simulink library "INT_Fans_trq"  (R2016b)
settings: Solver=VariableStepAuto  StartTime=0.0  StopTime=10.0  RelTol=1e-3
settings Model: Creator=xinchangran  LastModifiedBy=xinchangran

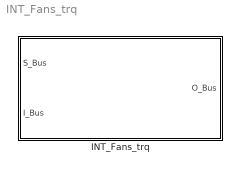
== system INT_Fans_trq ==
  INT_Fans_trq : Subsystem

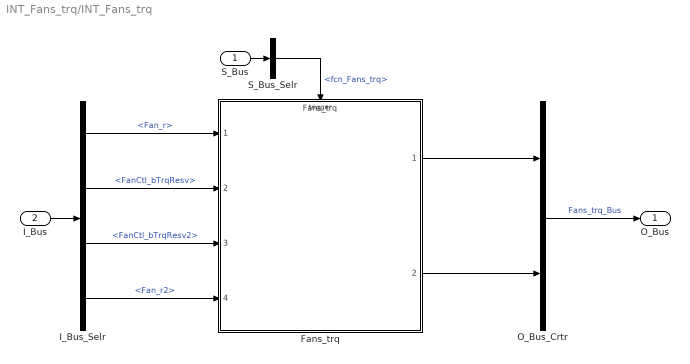
== system INT_Fans_trq/INT_Fans_trq ==
  S_Bus : Inport
  I_Bus : Inport  Port=2
  Fans_trq : ModelReference  ModelNameDialog=Fans_trq  SimulationMode=Normal  ModelReferenceVersion=1.16  TriggerPortName=function  TriggerPortTriggerType=function-call  TriggerPortStatesWhenEnabling=held
  I_Bus_Selr : BusSelector  OutputSignals=Fan_r,FanCtl_bTrqResv,FanCtl_bTrqResv2,Fan_r2
  O_Bus_Crtr : BusCreator  Inputs=2
  S_Bus_Selr : BusSelector  OutputSignals=fcn_Fans_trq
  O_Bus : Outport
  wires:
  S_Bus_Selr/1 -> Fans_trq/Trigger  "<fcn_Fans_trq>"
  S_Bus/1 -> S_Bus_Selr/1
  I_Bus/1 -> I_Bus_Selr/1
  I_Bus_Selr/1 -> Fans_trq/1  "<Fan_r>"
  I_Bus_Selr/2 -> Fans_trq/2  "<FanCtl_bTrqResv>"
  I_Bus_Selr/3 -> Fans_trq/3  "<FanCtl_bTrqResv2>"
  I_Bus_Selr/4 -> Fans_trq/4  "<Fan_r2>"
  O_Bus_Crtr/1 -> O_Bus/1  "Fans_trq_Bus"
  Fans_trq/1 -> O_Bus_Crtr/1
  Fans_trq/2 -> O_Bus_Crtr/2
